simulink model "SecRwRtStHdrstUpwdDnwdCtrl"  (R2018b)
settings: Solver=FixedStepDiscrete  StartTime=0.0  StopTime=10.0  FixedStep=0.01  RelTol=1e-3
undefined symbols (not defined in the file or in its folder): KeSMSuMdMotFinshdTm_Val, KeSMSuMdRetryTm1_Val, KeSMSuModeReqDurgTm_Val, KeSMSwSecRwRtStHdrstUpwdDnwdEnTrigBitMask_Val
libraries: StCtrlLib x1
settings Model: Creator=sn2xws  LastModifiedBy=sn2xws
settings DataIOCC: SaveFormat=StructureWithTime
settings OptimizationCC: DefaultParameterBehavior=Inlined  EnhancedBackFolding=on  PassReuseOutputArgsAs=Individual arguments  ZeroExternalMemoryAtStartup=off  ZeroInternalMemoryAtStartup=off  OptimizeBlockOrder=speed  DifferentSizesBufferReuse=on  OptimizationCustomize=off
settings DebuggingCC: ParameterTunabilityLossMsg=error
settings ModelReferenceCC: ModelReferenceNumInstancesAllowed=Single
settings SFSimCC: MATLABDynamicMemAlloc=off
settings RTWCC: SystemTargetFile=autosar.tlc  GenCodeOnly=on  TemplateMakefile=ert_default_tmf  Description=AUTOSAR  GenerateReport=on  IncludeHyperlinkInReport=on  LaunchReport=on  GenerateTraceInfo=on  GenerateTraceReport=on  GenerateTraceReportSl=on  GenerateTraceReportSf=on  GenerateTraceReportEml=on
settings CodeAppCC: ForceParamTrailComments=on  IgnoreCustomStorageClasses=off  OperatorAnnotations=on  SimulinkDataObjDesc=on  SFDataObjDesc=on  InsertBlockDesc=on
settings STFCustomTargetCC: TargetLangStandard=C99 (ISO)  MultiwordLength=256  ParMdlRefBuildCompliant=on  CompOptLevelCompliant=on  IncludeMdlTerminateFcn=off  CombineOutputUpdateFcns=on  SuppressErrorStatus=on  ERTCustomFileBanners=on  SupportNonFinite=off  SupportComplex=off  SupportContinuousTime=off  SupportNonInlinedSFcns=off  RemoveResetFunc=on  MATLABClassNameForMDSCustomization=Simulink.SoftwareTarget.ERTCustomization  AutosarCompliant=on  UseToolchainInfoCompliant=on  LookupTableObjectStructAxisOrder=2,1,3,4,...  LUTObjectStructOrderEvenSpacing=Size,Table,Breakpoints  SystemTargetFile=autosar.tlc
settings ERTTargetCC: TargetLangStandard=C99 (ISO)  ConcurrentExecutionCompliant=off  IncludeMdlTerminateFcn=off  SuppressErrorStatus=on  SupportNonFinite=off  SupportComplex=off  ModelStepFunctionPrototypeControlCompliant=off  CPPClassGenCompliant=off  AutosarCompliant=on  LookupTableObjectStructAxisOrder=2,1,3,4,...  LUTObjectStructOrderEvenSpacing=Size,Table,Breakpoints  InlinedParameterPlacement=NonHierarchical  ERTCustomFileTemplate=example_file_process.tlc  ERTFilePackagingFormat=Compact

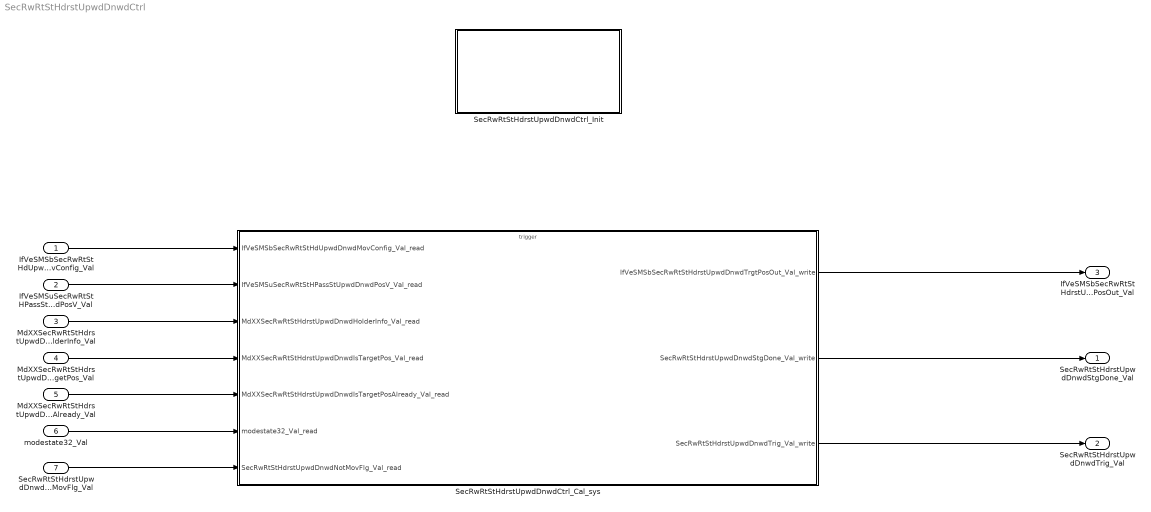
== system SecRwRtStHdrstUpwdDnwdCtrl ==
  IfVeSMSbSecRwRtStHdUpwdDnwdMovConfig_Val : Inport  OutDataTypeStr=boolean  PortDimensions=1
  IfVeSMSuSecRwRtStHPassStUpwdDnwdPosV_Val : Inport  Port=2  OutDataTypeStr=boolean  PortDimensions=1
  MdXXSecRwRtStHdrstUpwdDnwdHolderInfo_Val : Inport  Port=3  OutDataTypeStr=uint32  PortDimensions=1
  MdXXSecRwRtStHdrstUpwdDnwdIsTargetPos_Val : Inport  Port=4  OutDataTypeStr=uint32  PortDimensions=1
  MdXXSecRwRtStHdrstUpwdDnwdIsTargetPosAlready_Val : Inport  Port=5  OutDataTypeStr=uint32  PortDimensions=1
  modestate32_Val : Inport  Port=6  OutDataTypeStr=uint32  PortDimensions=1
  SecRwRtStHdrstUpwdDnwdNotMovFlg_Val : Inport  Port=7  OutDataTypeStr=boolean  PortDimensions=1
  SecRwRtStHdrstUpwdDnwdCtrl_Cal_sys : Subsystem
  SecRwRtStHdrstUpwdDnwdCtrl_Init : Subsystem
  SecRwRtStHdrstUpwdDnwdStgDone_Val : Outport  OutDataTypeStr=boolean  PortDimensions=1
  SecRwRtStHdrstUpwdDnwdTrig_Val : Outport  Port=2  OutDataTypeStr=boolean  PortDimensions=1
  IfVeSMSbSecRwRtStHdrstUpwdDnwdTrgtPosOut_Val : Outport  Port=3  OutDataTypeStr=boolean  PortDimensions=1
  wires:
  IfVeSMSbSecRwRtStHdUpwdDnwdMovConfig_Val/1 -> SecRwRtStHdrstUpwdDnwdCtrl_Cal_sys/1(IfVeSMSbSecRwRtStHdUpwdDnwdMovConfig_Val_read)
  IfVeSMSuSecRwRtStHPassStUpwdDnwdPosV_Val/1 -> SecRwRtStHdrstUpwdDnwdCtrl_Cal_sys/2(IfVeSMSuSecRwRtStHPassStUpwdDnwdPosV_Val_read)
  MdXXSecRwRtStHdrstUpwdDnwdHolderInfo_Val/1 -> SecRwRtStHdrstUpwdDnwdCtrl_Cal_sys/3(MdXXSecRwRtStHdrstUpwdDnwdHolderInfo_Val_read)
  MdXXSecRwRtStHdrstUpwdDnwdIsTargetPos_Val/1 -> SecRwRtStHdrstUpwdDnwdCtrl_Cal_sys/4(MdXXSecRwRtStHdrstUpwdDnwdIsTargetPos_Val_read)
  MdXXSecRwRtStHdrstUpwdDnwdIsTargetPosAlready_Val/1 -> SecRwRtStHdrstUpwdDnwdCtrl_Cal_sys/5(MdXXSecRwRtStHdrstUpwdDnwdIsTargetPosAlready_Val_read)
  modestate32_Val/1 -> SecRwRtStHdrstUpwdDnwdCtrl_Cal_sys/6(modestate32_Val_read)
  SecRwRtStHdrstUpwdDnwdNotMovFlg_Val/1 -> SecRwRtStHdrstUpwdDnwdCtrl_Cal_sys/7(SecRwRtStHdrstUpwdDnwdNotMovFlg_Val_read)
  SecRwRtStHdrstUpwdDnwdCtrl_Cal_sys/1(IfVeSMSbSecRwRtStHdrstUpwdDnwdTrgtPosOut_Val_write) -> IfVeSMSbSecRwRtStHdrstUpwdDnwdTrgtPosOut_Val/1
  SecRwRtStHdrstUpwdDnwdCtrl_Cal_sys/2(SecRwRtStHdrstUpwdDnwdStgDone_Val_write) -> SecRwRtStHdrstUpwdDnwdStgDone_Val/1
  SecRwRtStHdrstUpwdDnwdCtrl_Cal_sys/3(SecRwRtStHdrstUpwdDnwdTrig_Val_write) -> SecRwRtStHdrstUpwdDnwdTrig_Val/1

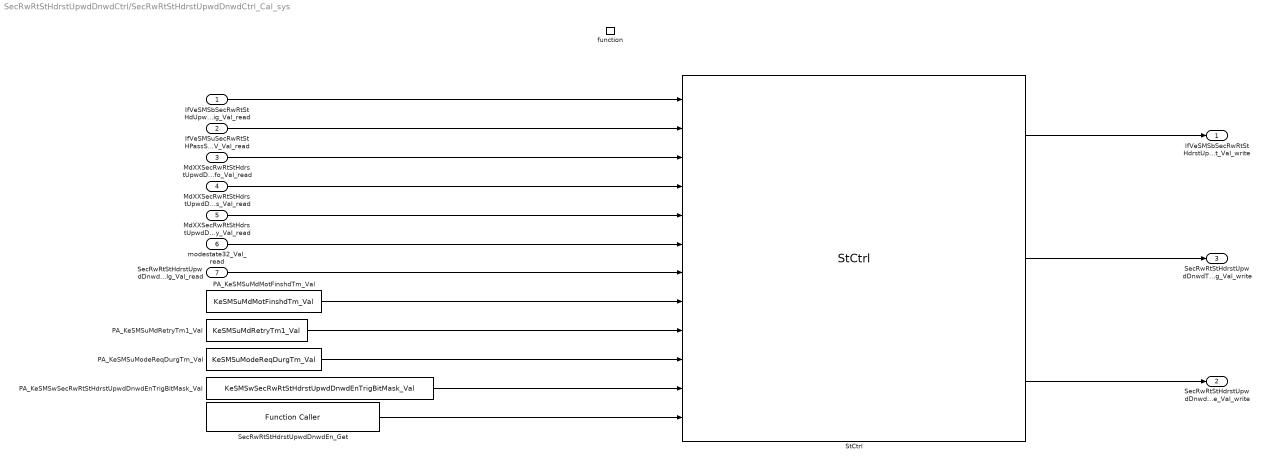
== system SecRwRtStHdrstUpwdDnwdCtrl/SecRwRtStHdrstUpwdDnwdCtrl_Cal_sys ==
  IfVeSMSbSecRwRtStHdUpwdDnwdMovConfig_Val_read : Inport
  IfVeSMSuSecRwRtStHPassStUpwdDnwdPosV_Val_read : Inport  Port=2
  MdXXSecRwRtStHdrstUpwdDnwdHolderInfo_Val_read : Inport  Port=3
  MdXXSecRwRtStHdrstUpwdDnwdIsTargetPos_Val_read : Inport  Port=4
  MdXXSecRwRtStHdrstUpwdDnwdIsTargetPosAlready_Val_read : Inport  Port=5
  modestate32_Val_read : Inport  Port=6
  SecRwRtStHdrstUpwdDnwdNotMovFlg_Val_read : Inport  Port=7
  function : TriggerPort  TriggerType=function-call  IsSimulinkFunction=on  FunctionName=SecRwRtStHdrstUpwdDnwdCtrl_Cal  VariantControl=(inherit)
  PA_KeSMSuMdMotFinshdTm_Val : Constant  Value=KeSMSuMdMotFinshdTm_Val
  PA_KeSMSuMdRetryTm1_Val : Constant  Value=KeSMSuMdRetryTm1_Val
  PA_KeSMSuModeReqDurgTm_Val : Constant  Value=KeSMSuModeReqDurgTm_Val
  PA_KeSMSwSecRwRtStHdrstUpwdDnwdEnTrigBitMask_Val : Constant  Value=KeSMSwSecRwRtStHdrstUpwdDnwdEnTrigBitMask_Val
  SecRwRtStHdrstUpwdDnwdEn_Get : FunctionCaller  FunctionPrototype=data = SecRwRtStHdrstUpwdDnwdEn_Get()  OutputArgumentSpecifications=uint32(1)
  StCtrl : StCtrlLib/StCtrl  SystemSampleTime=-1
  IfVeSMSbSecRwRtStHdrstUpwdDnwdTrgtPosOut_Val_write : Outport
      settings: EnsureOutportIsVirtual=on
  SecRwRtStHdrstUpwdDnwdStgDone_Val_write : Outport  Port=2
      settings: EnsureOutportIsVirtual=on
  SecRwRtStHdrstUpwdDnwdTrig_Val_write : Outport  Port=3
      settings: EnsureOutportIsVirtual=on
  wires:
  StCtrl/3 -> SecRwRtStHdrstUpwdDnwdStgDone_Val_write/1
  StCtrl/1 -> IfVeSMSbSecRwRtStHdrstUpwdDnwdTrgtPosOut_Val_write/1
  StCtrl/2 -> SecRwRtStHdrstUpwdDnwdTrig_Val_write/1
  PA_KeSMSwSecRwRtStHdrstUpwdDnwdEnTrigBitMask_Val/1 -> StCtrl/11
  SecRwRtStHdrstUpwdDnwdEn_Get/1 -> StCtrl/12
  PA_KeSMSuMdMotFinshdTm_Val/1 -> StCtrl/8
  PA_KeSMSuModeReqDurgTm_Val/1 -> StCtrl/10
  PA_KeSMSuMdRetryTm1_Val/1 -> StCtrl/9
  IfVeSMSbSecRwRtStHdUpwdDnwdMovConfig_Val_read/1 -> StCtrl/1
  IfVeSMSuSecRwRtStHPassStUpwdDnwdPosV_Val_read/1 -> StCtrl/2
  MdXXSecRwRtStHdrstUpwdDnwdHolderInfo_Val_read/1 -> StCtrl/3
  MdXXSecRwRtStHdrstUpwdDnwdIsTargetPos_Val_read/1 -> StCtrl/4
  MdXXSecRwRtStHdrstUpwdDnwdIsTargetPosAlready_Val_read/1 -> StCtrl/5
  modestate32_Val_read/1 -> StCtrl/6
  SecRwRtStHdrstUpwdDnwdNotMovFlg_Val_read/1 -> StCtrl/7

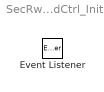
== system SecRwRtStHdrstUpwdDnwdCtrl/SecRwRtStHdrstUpwdDnwdCtrl_Init ==
  Event Listener : EventListener  EventName=reset
